simulink model "Final_project_TEMPLATE"  (R2015b)
settings: Solver=FixedStepDiscrete  StartTime=0.0  StopTime=10.0  RelTol=1e-3
InitFcn:
  | parameters
values from neighbouring files (symbols this model uses):
  Ak = 100    [parameters.m]
  b = 100    [parameters.m]
  dc_sathigh = .76    (= 0.76)    [parameters.m]
  dc_satlow = .24    (= 0.24)    [parameters.m]
  dT = 0.01    [parameters.m]
  H = 20    [parameters.m]
  L1 = 1.6    [parameters.m]
  L2 = 0.8    [parameters.m]
  m = 2000    [parameters.m]
  n_desired = 0    [parameters.m]
  pot_gain = 1    [parameters.m]
  pot_offset = 512    [parameters.m]
  R = 1/5    (= 0.2)    [parameters.m]
  S_Kd1 = .045    (= 0.045)    [parameters.m]
  S_Kd2 = 80    [parameters.m]
  S_Ki2 = 0.0001    [parameters.m]
  S_Kp1 = 0.45    [parameters.m]
  S_Kp2 = 600    [parameters.m]
  t2d = 2*pi/4000    (= 0.00157079632679)    [parameters.m]
  V_Ki = 50    [parameters.m]
  V_Kp = 5000    [parameters.m]
undefined symbols (not defined in the file or in its folder): A10, A13, A14, AN0, AN12, B, B13, B4, B6, C6, D, D11, D4, DiscIntNeverNeededParam, F15, F3, F4, G4, H4, L3, M14, N15, PA10, PA11, PA12, PA13, PA14, PA5, PA6, PA7, PA8, PA9, PB10, PB7, PC11, PC12, PC13, PC6, PD11, R10, R16, R5, R8
libraries: Conv_Lib x54, rappid_564xl_ec_toolbox x37, Veh_Sim x9, simulink x2, U_of_M_5643_blockset x1
(part 2 of 2)

== system Final_project_TEMPLATE/High Level Design/ACC/Speed Ctrl/PI/My Discrete Integrator ==
  X_dot : Inport
  Gain : Gain  Gain=dT  SaturateOnIntegerOverflow=on  OutDataTypeStr=Inherit: Same as input  ParamDataTypeStr=Inherit: Same as input
  Sum : Sum  Inputs=|++  SaturateOnIntegerOverflow=on  InputSameDT=on  OutDataTypeStr=Inherit: Same as first input
  Unit Delay : UnitDelay  SampleTime=-1
  X : Outport
  wires:
  Gain/1 -> Sum/1
  X_dot/1 -> Gain/1
  Sum/1 -> Unit Delay/1
  Unit Delay/1 -> Sum/2, X/1

== stateflow chart Final_project_TEMPLATE/High Level Design/ACC/ACC State Logic/En_choice ==
  state PositionControl_
    entry: en_man=false;
    en_vel = false;
    en_pos = true;
  state Manual__
    entry: en_man=true;
    en_vel = false;
    en_pos = false;
  state VelocityControl_
    entry: en_man=false ;
    en_vel = true;
    en_pos = false;
  Manual__ -> VelocityControl_ [order 1] : [(Man_en==0) &((Usi>Us+1) | (Si-Sm>H) | (Si==Sm))]
  Manual__ -> PositionControl_ [order 2] : [(Man_en==0) & ((Usi<=Us-1) & (Si-Sm<=H))&(Si~=Sm)]
  VelocityControl_ -> PositionControl_ [order 2] : [(Man_en==0) & ((Usi<=Us-1) & (Si-Sm<=H))&(Si~=Sm)]
  (default) -> Manual__
  VelocityControl_ -> Manual__ [order 1] : [Man_en==1]
  PositionControl_ -> VelocityControl_ [order 2] : [(Man_en==0) &((Usi>Us+1) | (Si-Sm>H) | (Si==Sm))]
  PositionControl_ -> Manual__ [order 1] : [Man_en==1]
  data: en_man output boolean; en_vel output boolean; en_pos output boolean; Man_en input; Usi input; Us input; H input; Si input; Sm input
